simulink model "vibration_simulink"  (R2018a)
settings: Solver=ode1  StartTime=0.0  StopTime=inf  RelTol=1e-3  EnableMultiTasking=on
libraries: arduinolib x2, simulink x2, dspstat3 x2, dspxfrm3 x1
settings Model: SimulationMode=external  ExtModeTrigDuration=2  Creator=chows  LastModifiedBy=chows
settings OptimizationCC: EnhancedBackFolding=on  PassReuseOutputArgsAs=Individual arguments  MaxStackSize=64  OptimizeBlockOrder=speed  DifferentSizesBufferReuse=on  OptimizationCustomize=off
settings DebuggingCC: ParameterTunabilityLossMsg=error
settings HardwareCC: ProdBitPerInt=16  ProdBitPerPointer=16  ProdBitPerSizeT=16  ProdBitPerPtrDiffT=16  ProdLargestAtomicFloat=None  ProdWordSize=8  ProdHWDeviceType=Atmel->AVR
settings SFSimCC: MATLABDynamicMemAlloc=off
settings RTWCC: SystemTargetFile=ert.tlc  HardwareBoard=Arduino Mega 2560  TLCOptions=-aInlineSetEventsForThisBaseRateFcn=TLC_FALSE -aSuppressMultiTaskScheduler=TLC_FALSE -aRateBasedStepFcn=1  TemplateMakefile=ert_default_tmf  GenerateReport=on  Toolchain=Arduino AVR  BuildConfiguration=Faster Runs  IncludeHyperlinkInReport=on  LaunchReport=on  GenerateTraceInfo=on  GenerateTraceReport=on  GenerateTraceReportSl=on  GenerateTraceReportSf=on  GenerateTraceReportEml=on
settings CodeAppCC: ForceParamTrailComments=on  IgnoreCustomStorageClasses=off  OperatorAnnotations=on  SimulinkDataObjDesc=on  SFDataObjDesc=on  InsertBlockDesc=on
settings ERTTargetCC: SupportContinuousTime=on  SupportVariableSizeSignals=on

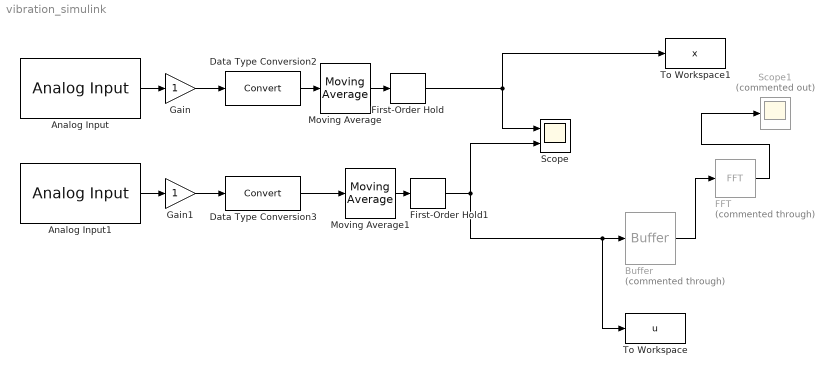
== system vibration_simulink ==
  Analog Input : arduinolib/Analog Input  pinNumber=4  ReadResultsOnly=off  ConversionTriggerSource=Software  ExternalTriggerType=uint32(0)  OutputDataType=uint16  EnableConversionCompleteNotify=off  EnableOuputStatus=off  SampleTime=0.001  blockPlatform=arduino
  Analog Input1 : arduinolib/Analog Input  pinNumber=5  ReadResultsOnly=off  ConversionTriggerSource=Software  ExternalTriggerType=uint32(0)  OutputDataType=uint16  EnableConversionCompleteNotify=off  EnableOuputStatus=off  SampleTime=0.001  blockPlatform=arduino
  Buffer : Buffer  Commented=through  N=128  OutputFrames=off
  Data Type Conversion2 : DataTypeConversion
  Data Type Conversion3 : DataTypeConversion
  FFT : dspxfrm3/FFT  Commented=through  FFTImplementation=Auto  CompMethod=Table lookup  TableOpt=NEW  TableOptActive=Speed  BitRevOrder=off  Normalize=off  InheritFFTLength=off  FFTLength=256  WrapInput=on  roundingMode=Floor  overflowMode=off  firstCoeffDataTypeStr=Inherit: Same word length as input  firstCoeffLastDataTypeStr=Inherit: Same word length as input  outputMin=[]  outputMax=[]
  First-Order Hold : simulink/Discrete/First-Order Hold  DisableCoverage=on  Ts=0.001
      settings: SourceProductName=Simulink  SourceProductBaseCode=SL
  First-Order Hold1 : simulink/Discrete/First-Order Hold  DisableCoverage=on  Ts=0.001
      settings: SourceProductName=Simulink  SourceProductBaseCode=SL
  Gain : Gain
  Gain1 : Gain
  Moving Average : dspstat3/Moving Average  Method=Sliding window  ForgettingFactorPort=off  SpecifyWindowLength=on  WindowLength=50  ForgettingFactor=0.9  SimulateUsing=Code generation
  Moving Average1 : dspstat3/Moving Average  Method=Sliding window  ForgettingFactorPort=off  SpecifyWindowLength=on  WindowLength=50  ForgettingFactor=0.9  SimulateUsing=Code generation
  Scope : Scope  NumInputPorts=2
  Scope1 : Scope  Commented=on
  To Workspace : ToWorkspace  VariableName=u  SaveFormat=Timeseries  SampleTime=-1
  To Workspace1 : ToWorkspace  VariableName=x  SaveFormat=Timeseries  SampleTime=-1
  wires:
  Analog Input1/1 -> Gain1/1
  Analog Input/1 -> Gain/1
  First-Order Hold1/1 -> To Workspace/1, Buffer/1, Scope/2
  FFT/1 -> Scope1/1
  Buffer/1 -> FFT/1
  First-Order Hold/1 -> To Workspace1/1, Scope/1
  Gain/1 -> Data Type Conversion2/1
  Gain1/1 -> Data Type Conversion3/1
  Moving Average/1 -> First-Order Hold/1
  Moving Average1/1 -> First-Order Hold1/1
  Data Type Conversion2/1 -> Moving Average/1
  Data Type Conversion3/1 -> Moving Average1/1
